simulink subsystem "SenalizacionLuces"  (R2023b)
settings: Solver=VariableStepAuto  StartTime=0.0  StopTime=10.0  RelTol=1e-3
libraries: simulink x2
settings Model: Creator=Andrés  LastModifiedBy=Andrés

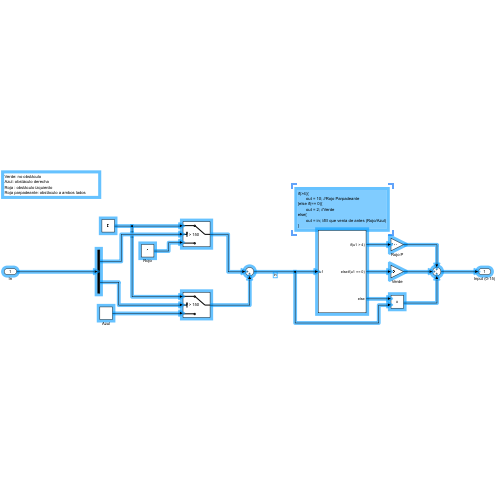
[thumbnail: Simulink's stored preview of the top-level diagram]
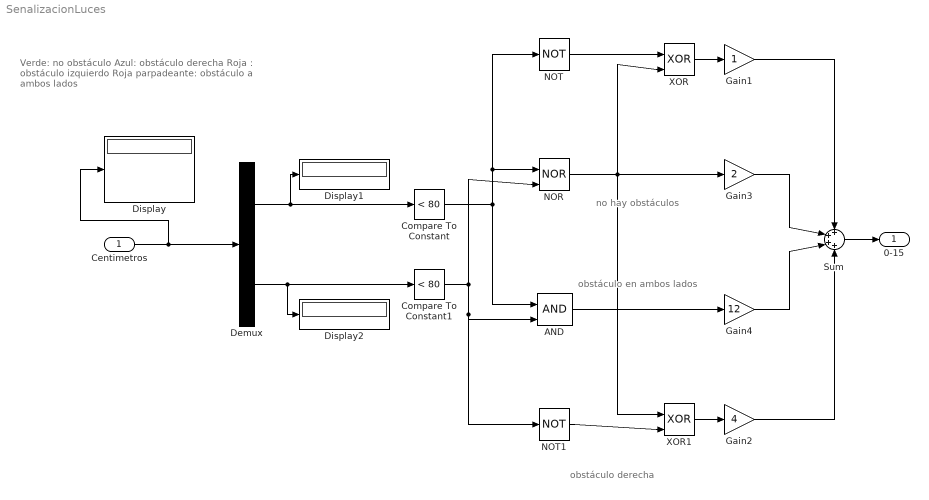
== system SenalizacionLuces ==
  note: obstáculo derecha
  note: obstáculo en ambos lados
  note: no hay obstáculos
  note: Verde: no obstáculo
      | Azul: obstáculo derecha
      | Roja : obstáculo izquierdo
      | Roja parpadeante: obstáculo a ambos lados
  Centimetros : Inport
  AND : Logic  IconShape=distinctive  AllPortsSameDT=off  OutDataTypeStr=boolean
  Compare To Constant : simulink/Logic and Bit Operations/Compare To Constant  relop=<  const=80  OutDataTypeStr=boolean
  Compare To Constant1 : simulink/Logic and Bit Operations/Compare To Constant  relop=<  const=80  OutDataTypeStr=boolean
  Demux : Demux  Outputs=2
  Display : Display
  Display1 : Display
  Display2 : Display
  Gain1 : Gain
  Gain2 : Gain  Gain=4
  Gain3 : Gain  Gain=2
  Gain4 : Gain  Gain=12
  NOR : Logic  Operator=NOR  IconShape=distinctive  AllPortsSameDT=off  OutDataTypeStr=boolean
  NOT : Logic  Operator=NOT  IconShape=distinctive  AllPortsSameDT=off  OutDataTypeStr=boolean
  NOT1 : Logic  Operator=NOT  IconShape=distinctive  AllPortsSameDT=off  OutDataTypeStr=boolean
  Sum : Sum  Inputs=++++
  XOR : Logic  Operator=XOR  IconShape=distinctive  AllPortsSameDT=off  OutDataTypeStr=boolean
  XOR1 : Logic  Operator=XOR  IconShape=distinctive  AllPortsSameDT=off  OutDataTypeStr=boolean
  0-15 : Outport
  wires:
  NOT1/1 -> XOR1/2
  Demux/1 -> Compare To Constant/1, Display1/1
  Gain2/1 -> Sum/4
  Gain4/1 -> Sum/3
  XOR1/1 -> Gain2/1
  NOR/1 -> XOR/2, XOR1/1, Gain3/1
  NOT/1 -> XOR/1
  AND/1 -> Gain4/1
  Gain3/1 -> Sum/2
  Sum/1 -> 0-15/1
  Compare To Constant1/1 -> NOR/2, NOT1/1, AND/2
  Centimetros/1 -> Demux/1, Display/1
  Gain1/1 -> Sum/1
  Compare To Constant/1 -> NOR/1, NOT/1, AND/1
  Demux/2 -> Compare To Constant1/1, Display2/1
  XOR/1 -> Gain1/1
